simulink model "DesignDCMotorUsingPID"  (R2017a)
settings: Solver=ode45  StartTime=0.0  StopTime=10.0  RelTol=1e-3  EnableMultiTasking=on
values from neighbouring files (symbols this model uses):
  b = 3.1831E-4    (= 0.00031831)    [DesignDCMotorUsingPIDrlocusBode.m]    (also in DiscreteDesignandEquivalent.m; bode_mcode.m; exceldata.m = b'; il_zom_hae_byungsina.m)
  J = 52E-7    (= 5.2e-06)    [DesignDCMotorUsingPIDrlocusBode.m]    (also in DiscreteDesignandEquivalent.m; bode_mcode.m; il_zom_hae_byungsina.m; rlocus_mcode.m)
  K = 0.0245    [DesignDCMotorUsingPIDrlocusBode.m]    (also in DiscreteDesignandEquivalent.m; bode_mcode.m; il_zom_hae_byungsina.m; pid_mcode.m)
  L = 10    [AEB_TTC_test.m]    (also in DesignDCMotorUsingPIDrlocusBode.m = 0.0024; DiscreteDesignandEquivalent.m = 0.0024; bode_mcode.m = 0.0024; errorvsstepsize.m = [H' D' E']')
  R = 1.8    [DesignDCMotorUsingPIDrlocusBode.m]    (also in DiscreteDesignandEquivalent.m; RCCircuit_data_plot2.m = 1; bode_mcode.m; il_zom_hae_byungsina.m)
  s = tf('s')    [DesignDCMotorUsingPIDrlocusBode.m]    (also in DiscreteDesignExample.m; DiscreteDesignandEquivalent.m; DiscreteEquivalentExample.m; DiscreteTest.m)
settings Model: Creator=gyurse  LastModifiedBy=edward
settings DataIOCC: LimitDataPoints=on  SaveFormat=Array
settings OptimizationCC: LifeSpan=inf
settings DebuggingCC: UnderspecifiedInitializationDetection=Classic  MergeDetectMultiDrivingBlocksExec=none  SolverPrmCheckMsg=warning  SFUnexpectedBacktrackingDiag=warning  SFNoUnconditionalDefaultTransitionDiag=warning  SFExecutionAtInitializationDiag=none
settings HardwareCC: ProdBitPerPointer=32  ProdBitPerSizeT=32  ProdBitPerPtrDiffT=32  ProdLargestAtomicFloat=None  ProdIntDivRoundTo=Undefined  ProdEndianess=Unspecified  ProdWordSize=32  ProdHWDeviceType=32-bit Generic
settings ModelReferenceCC: PropagateSignalLabelsOutOfModel=off
settings GRTTargetCC: TargetLangStandard=C89/C90 (ANSI)  GeneratePreprocessorConditionals=Disable all
settings ConfigComp: CovMetricSettings=dw  CovHtmlReporting=on  CovSaveCumulativeToWorkspaceVar=on  CovSaveSingleToWorkspaceVar=on  CovExternalEMLEnable=off

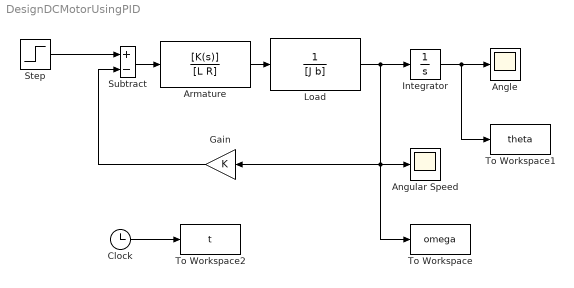
== system DesignDCMotorUsingPID ==
  "Angle " : Scope
  "Angular Speed " : Scope
  "Armature " : TransferFcn  Numerator=[K(s)]  Denominator=[L R]
  Clock : Clock
  Gain : Gain  Gain=K
  Integrator : Integrator
  "Load " : TransferFcn  Denominator=[J b]
  Step : Step  SampleTime=0
  Subtract : Sum  Inputs=+-
  To Workspace : ToWorkspace  VariableName=omega  SaveFormat=Timeseries  SampleTime=-1
  To Workspace1 : ToWorkspace  VariableName=theta  SaveFormat=Timeseries  SampleTime=-1
  To Workspace2 : ToWorkspace  VariableName=t  SaveFormat=Timeseries  SampleTime=-1
  wires:
  Gain/1 -> Subtract/2
  Step/1 -> Subtract/1
  Subtract/1 -> "Armature "/1
  "Armature "/1 -> "Load "/1
  Clock/1 -> To Workspace2/1
  Integrator/1 -> To Workspace1/1, "Angle "/1
  "Load "/1 -> To Workspace/1, "Angular Speed "/1, Gain/1, Integrator/1
